simulink model "p1g2"  (R2018a)
settings: Solver=VariableStepAuto  StartTime=0.0  StopTime=1  RelTol=1e-3
values from neighbouring files (symbols this model uses):
  C = 10    [ef.m]
  J = 0.006    [ef.m]
  Ka = 1    [ef.m]
  Kb = 0.0706    [ef.m]
  Km = 10    [ef.m]
  R = 0.1    [ef.m]
settings Model: Creator=carma  LastModifiedBy=carma

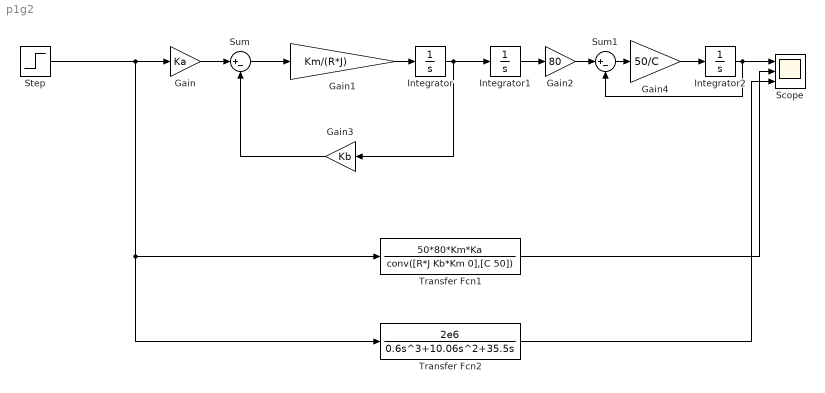
== system p1g2 ==
  Gain : Gain  Gain=Ka
  Gain1 : Gain  Gain=Km/(R*J)
  Gain2 : Gain  Gain=80
  Gain3 : Gain  Gain=Kb
  Gain4 : Gain  Gain=50/C
  Integrator : Integrator
  Integrator1 : Integrator
  Integrator2 : Integrator
  Scope : Scope  NumInputPorts=3
  Step : Step  Time=0  SampleTime=0
  Sum : Sum  Inputs=|+-
  Sum1 : Sum  Inputs=|+-
  Transfer Fcn1 : TransferFcn  Numerator=50*80*Km*Ka  Denominator=conv([R*J Kb*Km 0],[C 50])
  Transfer Fcn2 : TransferFcn  Numerator=2e6  Denominator="[0.6  10.06 35.5 0]"
  wires:
  Transfer Fcn1/1 -> Scope/2
  Gain3/1 -> Sum/2
  Integrator/1 -> Integrator1/1, Gain3/1
  Step/1 -> Gain/1, Transfer Fcn2/1, Transfer Fcn1/1
  Sum/1 -> Gain1/1
  Gain/1 -> Sum/1
  Gain1/1 -> Integrator/1
  Integrator1/1 -> Gain2/1
  Gain2/1 -> Sum1/1
  Sum1/1 -> Gain4/1
  Integrator2/1 -> Sum1/2, Scope/1
  Gain4/1 -> Integrator2/1
  Transfer Fcn2/1 -> Scope/3
